simulink model "ab"  (Simulink 10.0)
settings: Solver=ode45  StartTime=0.0  StopTime=1000  FixedStep=0.01  RelTol=1e-9  AbsTol=1e-12  EnableMultiTasking=on
settings Model: Creator=ec1099  LastModifiedBy=unknown
settings SolverCC: AutoScaleAbsTol=off
settings DataIOCC: SignalLoggingSaveFormat=ModelDataLogs  SaveOutput=off  SignalLogging=off  SaveTime=off
settings OptimizationCC: DefaultParameterBehavior=Inlined  ExpressionDepthLimit=2147483647  InitFltsAndDblsToZero=on  SimCompilerOptimization=on
settings DebuggingCC: FcnCallInpInsideContextMsg=warning  StateNameClashWarn=warning
settings ConfigComp: CovExternalEMLEnable=off

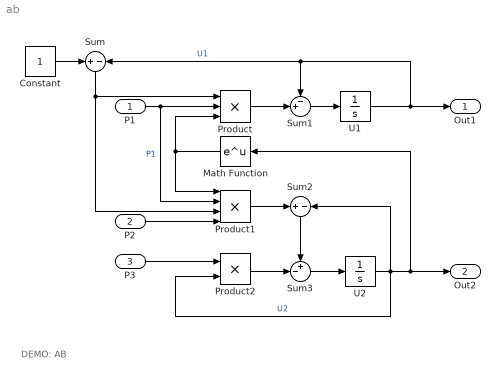
== system ab ==
  note: DEMO: AB
  P1 : Inport
  P2 : Inport  Port=2
  P3 : Inport  Port=3
  Constant : Constant
  Math Function : Math  SaturateOnIntegerOverflow=on
  Product : Product  Inputs=3  RndMeth=Zero
  Product1 : Product  Inputs=4  RndMeth=Zero
  Product2 : Product  RndMeth=Zero
  Sum : Sum  Inputs=+-
  Sum1 : Sum  Inputs=-+|
  Sum2 : Sum  Inputs=+-
  Sum3 : Sum  Inputs=+-|
  U1 : Integrator
  U2 : Integrator
  Out1 : Outport
  Out2 : Outport  Port=2
  wires:
  U1/1 -> Sum/2, Sum1/1, Out1/1  "U1"
  Constant/1 -> Sum/1
  U2/1 -> Sum2/2, Product2/2, Math Function/1, Out2/1  "U2"
  Math Function/1 -> Product/3, Product1/1
  P1/1 -> Product/2, Product1/2  "P1"
  Sum/1 -> Product/1, Product1/3
  Sum1/1 -> U1/1
  Product/1 -> Sum1/2
  P2/1 -> Product1/4
  Product1/1 -> Sum2/1
  P3/1 -> Product2/1
  Product2/1 -> Sum3/2
  Sum2/1 -> Sum3/1
  Sum3/1 -> U2/1
